simulink model "FOC"  (R2024b)
settings: Solver=ode4  StartTime=0.0  StopTime=0.5  FixedStep=Ts/10  RelTol=1e-3
InitFcn:
  | foc_param;
values from neighbouring files (symbols this model uses):
  B = 1e-6    (= 1e-06)    [foc_param.m]
  Iq_max = cast(Iq_max, FOC_dtype)    [foc_param.m]
  J = 0.4*1.829e-5    (= 7.316e-06)    [foc_param.m]
  Ki_dq = make_foc_parameter(Ki_dq_val, FOC_dtype, 'Id/Iq current PI integral gain',     'V/(A*s)')    [foc_param.m]
  Ki_w = make_foc_parameter(Ki_w_val,  FOC_dtype, 'Speed PI integral gain',             'A/rad')    [foc_param.m]
  Kp_dq = make_foc_parameter(Kp_dq_val, FOC_dtype, 'Id/Iq current PI proportional gain', 'V/A')    [foc_param.m]
  Kp_w = make_foc_parameter(Kp_w_val,  FOC_dtype, 'Speed PI proportional gain',         'A/(rad/s)')    [foc_param.m]
  p = 4    [foc_param.m]
  Spd_ref_tau = Kp_w_val/Ki_w_val    [foc_param.m]
  Ts = 1/20000    (= 5e-05)    [foc_param.m]
  Vmax = cast(Vmax,   FOC_dtype)    [foc_param.m]
undefined symbols (not defined in the file or in its folder): DiscIntNeverNeededParam
libraries: autolibpmsmexterior x1
settings Model: Creator=BitCore  LastModifiedBy=BitCore

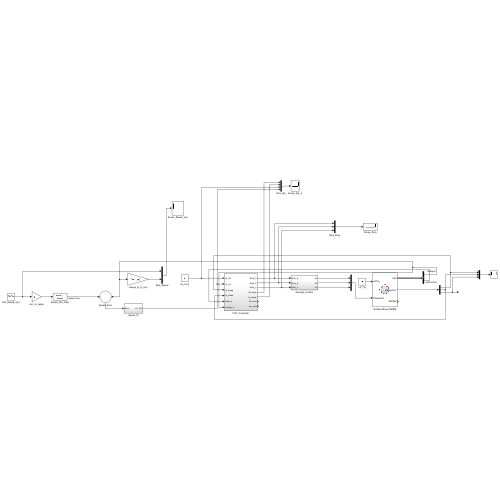
[thumbnail: Simulink's stored preview of the top-level diagram]
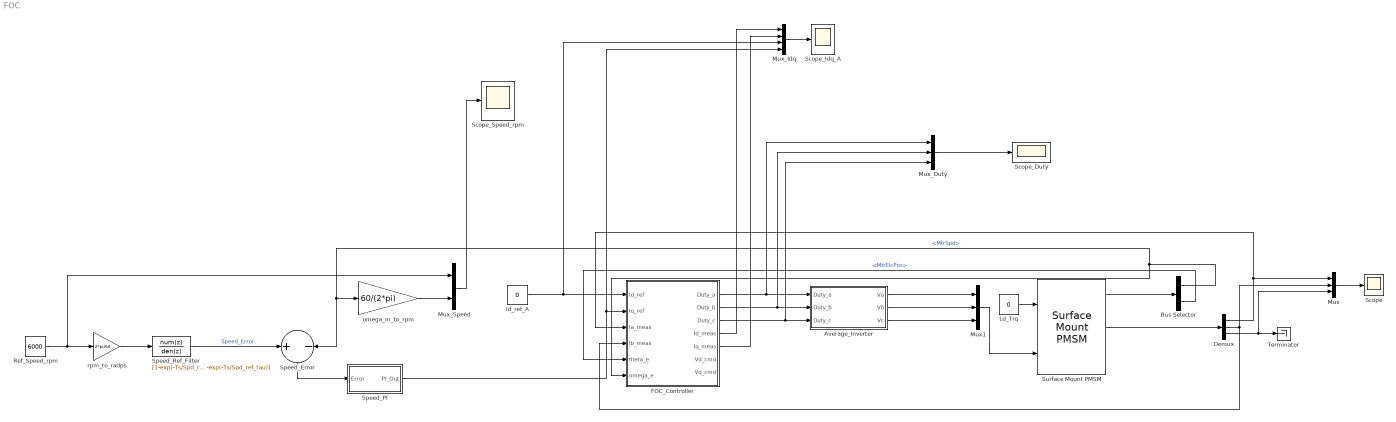
== system FOC ==
  Average_Inverter : Subsystem
  Bus Selector : BusSelector  OutputSignals=MtrSpd,MtrElcPos
  Demux : Demux  Outputs=3
  FOC_Controller : Subsystem
  Id_ref_A : Constant  Value=0
  Ld_Trq : Constant  Value=0
  Mux : Mux  Inputs=3
  Mux1 : Mux  Inputs=3
  Mux_Duty : Mux  Inputs=3
  Mux_Idq : Mux
  Mux_Speed : Mux  Inputs=2
  Ref_Speed_rpm : Constant  Value=6000
  Scope : Scope
  Scope_Duty : Scope
  Scope_Idq_A : Scope
  Scope_Speed_rpm : Scope
  Speed_Error : Sum  Inputs=+-
  Speed_PI : Subsystem
  Speed_Ref_Filter : DiscreteTransferFcn  Numerator=[1-exp(-Ts/Spd_ref_tau)]  Denominator=[1 -exp(-Ts/Spd_ref_tau)]  SampleTime=Ts
  Surface Mount PMSM : autolibpmsmexterior/Surface Mount PMSM  port_config=Torque  sim_type=Continuous  Ts=0.001  P=p  Rs=Rs  Ldq_=Ld  KConstText=Permanent flux linkage constant (lambda_pm):  lambda_pm=Lambda  Ke=159.9771  Kt=1.323  mechanical=[J B 0]  idq0=[0 0]  theta_init=0  omega_init=0  KConst=Lambda  lambda_pm_calc=Lambda  RefBlkName='autolibpmsmexterior/Surface Mount PMSM'  aMode=5  Ldq="[0.0017      0.0017]"
  Terminator : Terminator
  omega_m_to_rpm : Gain  Gain=60/(2*pi)
  rpm_to_radps : Gain  Gain=2*pi/60
  wires:
  Speed_Ref_Filter/1 -> Speed_Error/1  "Speed_Error"
  Mux_Duty/1 -> Scope_Duty/1
  Average_Inverter/3(Vc) -> Mux1/3
  FOC_Controller/1(Duty_a) -> Mux_Duty/1, Average_Inverter/1(Duty_a)
  Mux_Idq/1 -> Scope_Idq_A/1
  FOC_Controller/2(Duty_b) -> Mux_Duty/2, Average_Inverter/2(Duty_b)
  FOC_Controller/4(Id_meas) -> Mux_Idq/1
  Speed_PI/1(PI_Out) -> Mux_Idq/4, FOC_Controller/2(Iq_ref)
  Id_ref_A/1 -> Mux_Idq/3, FOC_Controller/1(Id_ref)
  Speed_Error/1 -> Speed_PI/1(Error)
  Demux/1 -> FOC_Controller/3(Ia_meas), Mux/1
  Average_Inverter/2(Vb) -> Mux1/2
  Bus Selector/1 -> Speed_Error/2, omega_m_to_rpm/1, FOC_Controller/6(omega_e)  "<MtrSpd>"
  FOC_Controller/3(Duty_c) -> Mux_Duty/3, Average_Inverter/3(Duty_c)
  FOC_Controller/5(Iq_meas) -> Mux_Idq/2
  Mux_Speed/1 -> Scope_Speed_rpm/1
  rpm_to_radps/1 -> Speed_Ref_Filter/1
  Ref_Speed_rpm/1 -> Mux_Speed/1, rpm_to_radps/1
  Demux/2 -> Mux/2, FOC_Controller/4(Ib_meas)
  omega_m_to_rpm/1 -> Mux_Speed/2
  Mux1/1 -> Surface Mount PMSM/2
  Average_Inverter/1(Va) -> Mux1/1
  Surface Mount PMSM/2 -> Demux/1
  Demux/3 -> Terminator/1, Mux/3
  Surface Mount PMSM/1 -> Bus Selector/1
  Mux/1 -> Scope/1
  Ld_Trq/1 -> Surface Mount PMSM/1
  Bus Selector/2 -> FOC_Controller/5(theta_e)  "<MtrElcPos>"

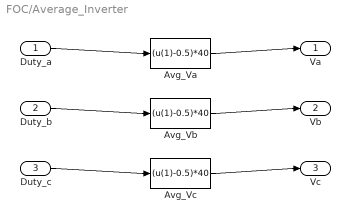
== system FOC/Average_Inverter ==
  Duty_a : Inport
  Duty_b : Inport  Port=2
  Duty_c : Inport  Port=3
  Avg_Va : Fcn  Expr=(u(1)-0.5)*40
  Avg_Vb : Fcn  Expr=(u(1)-0.5)*40
  Avg_Vc : Fcn  Expr=(u(1)-0.5)*40
  Va : Outport
  Vb : Outport  Port=2
  Vc : Outport  Port=3
  wires:
  Duty_a/1 -> Avg_Va/1
  Avg_Va/1 -> Va/1
  Duty_b/1 -> Avg_Vb/1
  Avg_Vb/1 -> Vb/1
  Duty_c/1 -> Avg_Vc/1
  Avg_Vc/1 -> Vc/1

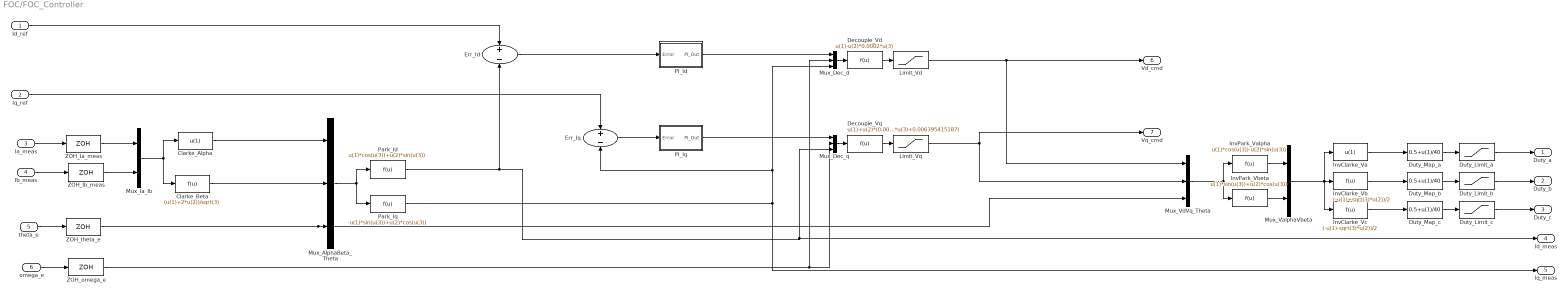
== system FOC/FOC_Controller ==
  Id_ref : Inport
  Iq_ref : Inport  Port=2
  Ia_meas : Inport  Port=3
  Ib_meas : Inport  Port=4
  theta_e : Inport  Port=5
  omega_e : Inport  Port=6
  Clarke_Alpha : Fcn  Expr=u(1)
  Clarke_Beta : Fcn  Expr=(u(1)+2*u(2))/sqrt(3)
  Decouple_Vd : Fcn  Expr=u(1)-u(2)*0.0002*u(3)
  Decouple_Vq : Fcn  Expr=u(1)+u(2)*(0.0002*u(3)+0.006395415187)
  Duty_Limit_a : Saturate  UpperLimit=1  LowerLimit=0
  Duty_Limit_b : Saturate  UpperLimit=1  LowerLimit=0
  Duty_Limit_c : Saturate  UpperLimit=1  LowerLimit=0
  Duty_Map_a : Fcn  Expr=0.5+u(1)/40
  Duty_Map_b : Fcn  Expr=0.5+u(1)/40
  Duty_Map_c : Fcn  Expr=0.5+u(1)/40
  Err_Id : Sum  Inputs=+-
  Err_Iq : Sum  Inputs=+-
  InvClarke_Va : Fcn  Expr=u(1)
  InvClarke_Vb : Fcn  Expr=(-u(1)+sqrt(3)*u(2))/2
  InvClarke_Vc : Fcn  Expr=(-u(1)-sqrt(3)*u(2))/2
  InvPark_Valpha : Fcn  Expr=u(1)*cos(u(3))-u(2)*sin(u(3))
  InvPark_Vbeta : Fcn  Expr=u(1)*sin(u(3))+u(2)*cos(u(3))
  Limit_Vd : Saturate  UpperLimit=Vmax  LowerLimit=-Vmax
  Limit_Vq : Saturate  UpperLimit=Vmax  LowerLimit=-Vmax
  Mux_AlphaBeta_Theta : Mux  Inputs=3
  Mux_Dec_d : Mux  Inputs=3
  Mux_Dec_q : Mux  Inputs=3
  Mux_Ia_Ib : Mux  Inputs=2
  Mux_ValphaVbeta : Mux  Inputs=2
  Mux_VdVq_Theta : Mux  Inputs=3
  PI_Id : Subsystem
  PI_Iq : Subsystem
  Park_Id : Fcn  Expr=u(1)*cos(u(3))+u(2)*sin(u(3))
  Park_Iq : Fcn  Expr=-u(1)*sin(u(3))+u(2)*cos(u(3))
  ZOH_Ia_meas : ZeroOrderHold  SampleTime=Ts
  ZOH_Ib_meas : ZeroOrderHold  SampleTime=Ts
  ZOH_omega_e : ZeroOrderHold  SampleTime=Ts
  ZOH_theta_e : ZeroOrderHold  SampleTime=Ts
  Duty_a : Outport
  Duty_b : Outport  Port=2
  Duty_c : Outport  Port=3
  Id_meas : Outport  Port=4
  Iq_meas : Outport  Port=5
  Vd_cmd : Outport  Port=6
  Vq_cmd : Outport  Port=7
  wires:
  Ia_meas/1 -> ZOH_Ia_meas/1
  Ib_meas/1 -> ZOH_Ib_meas/1
  theta_e/1 -> ZOH_theta_e/1
  omega_e/1 -> ZOH_omega_e/1
  ZOH_Ia_meas/1 -> Mux_Ia_Ib/1
  ZOH_Ib_meas/1 -> Mux_Ia_Ib/2
  Mux_Ia_Ib/1 -> Clarke_Alpha/1, Clarke_Beta/1
  Clarke_Alpha/1 -> Mux_AlphaBeta_Theta/1
  Clarke_Beta/1 -> Mux_AlphaBeta_Theta/2
  ZOH_theta_e/1 -> Mux_VdVq_Theta/3, Mux_AlphaBeta_Theta/3
  Mux_AlphaBeta_Theta/1 -> Park_Id/1, Park_Iq/1
  Id_ref/1 -> Err_Id/1
  Park_Id/1 -> Id_meas/1, Mux_Dec_q/3, Err_Id/2
  Iq_ref/1 -> Err_Iq/1
  Park_Iq/1 -> Iq_meas/1, Mux_Dec_d/3, Err_Iq/2
  Err_Id/1 -> PI_Id/1(Error)
  Err_Iq/1 -> PI_Iq/1(Error)
  PI_Id/1(PI_Out) -> Mux_Dec_d/1
  ZOH_omega_e/1 -> Mux_Dec_d/2, Mux_Dec_q/2
  PI_Iq/1(PI_Out) -> Mux_Dec_q/1
  Mux_Dec_d/1 -> Decouple_Vd/1
  Mux_Dec_q/1 -> Decouple_Vq/1
  Decouple_Vd/1 -> Limit_Vd/1
  Decouple_Vq/1 -> Limit_Vq/1
  Limit_Vd/1 -> Vd_cmd/1, Mux_VdVq_Theta/1
  Limit_Vq/1 -> Vq_cmd/1, Mux_VdVq_Theta/2
  Mux_VdVq_Theta/1 -> InvPark_Vbeta/1, InvPark_Valpha/1
  InvPark_Valpha/1 -> Mux_ValphaVbeta/1
  InvPark_Vbeta/1 -> Mux_ValphaVbeta/2
  Mux_ValphaVbeta/1 -> InvClarke_Vc/1, InvClarke_Va/1, InvClarke_Vb/1
  InvClarke_Va/1 -> Duty_Map_a/1
  Duty_Map_a/1 -> Duty_Limit_a/1
  Duty_Limit_a/1 -> Duty_a/1
  InvClarke_Vb/1 -> Duty_Map_b/1
  Duty_Map_b/1 -> Duty_Limit_b/1
  Duty_Limit_b/1 -> Duty_b/1
  InvClarke_Vc/1 -> Duty_Map_c/1
  Duty_Map_c/1 -> Duty_Limit_c/1
  Duty_Limit_c/1 -> Duty_c/1

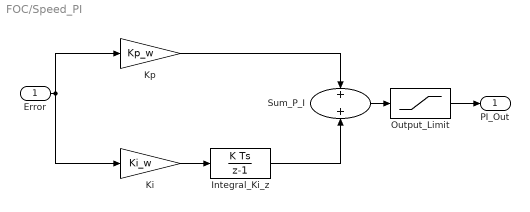
== system FOC/Speed_PI ==
  Error : Inport
  Integral_Ki_z : DiscreteIntegrator  SampleTime=Ts  LimitOutput=on  UpperSaturationLimit=Iq_max  LowerSaturationLimit=-Iq_max  ICPrevOutput=DiscIntNeverNeededParam  ICPrevScaledInput=DiscIntNeverNeededParam
  Ki : Gain  Gain=Ki_w
  Kp : Gain  Gain=Kp_w
  Output_Limit : Saturate  UpperLimit=Iq_max  LowerLimit=-Iq_max
  Sum_P_I : Sum
  PI_Out : Outport
  wires:
  Error/1 -> Kp/1, Ki/1
  Ki/1 -> Integral_Ki_z/1
  Kp/1 -> Sum_P_I/1
  Integral_Ki_z/1 -> Sum_P_I/2
  Sum_P_I/1 -> Output_Limit/1
  Output_Limit/1 -> PI_Out/1

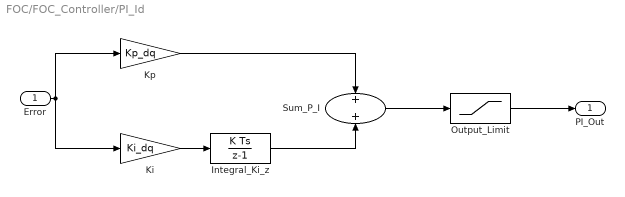
== system FOC/FOC_Controller/PI_Id ==
  Error : Inport
  Integral_Ki_z : DiscreteIntegrator  SampleTime=Ts  LimitOutput=on  UpperSaturationLimit=Vmax  LowerSaturationLimit=-Vmax  ICPrevOutput=DiscIntNeverNeededParam  ICPrevScaledInput=DiscIntNeverNeededParam
  Ki : Gain  Gain=Ki_dq
  Kp : Gain  Gain=Kp_dq
  Output_Limit : Saturate  UpperLimit=Vmax  LowerLimit=-Vmax
  Sum_P_I : Sum
  PI_Out : Outport
  wires:
  Error/1 -> Kp/1, Ki/1
  Ki/1 -> Integral_Ki_z/1
  Kp/1 -> Sum_P_I/1
  Integral_Ki_z/1 -> Sum_P_I/2
  Sum_P_I/1 -> Output_Limit/1
  Output_Limit/1 -> PI_Out/1

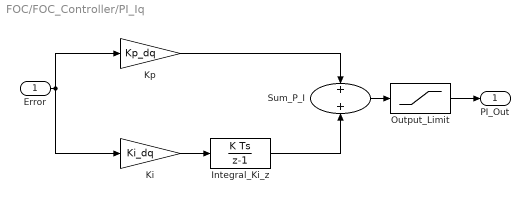
== system FOC/FOC_Controller/PI_Iq ==
  Error : Inport
  Integral_Ki_z : DiscreteIntegrator  SampleTime=Ts  LimitOutput=on  UpperSaturationLimit=Vmax  LowerSaturationLimit=-Vmax  ICPrevOutput=DiscIntNeverNeededParam  ICPrevScaledInput=DiscIntNeverNeededParam
  Ki : Gain  Gain=Ki_dq
  Kp : Gain  Gain=Kp_dq
  Output_Limit : Saturate  UpperLimit=Vmax  LowerLimit=-Vmax
  Sum_P_I : Sum
  PI_Out : Outport
  wires:
  Error/1 -> Kp/1, Ki/1
  Ki/1 -> Integral_Ki_z/1
  Kp/1 -> Sum_P_I/1
  Integral_Ki_z/1 -> Sum_P_I/2
  Sum_P_I/1 -> Output_Limit/1
  Output_Limit/1 -> PI_Out/1
